simulink library "csbenchlab_est"  (R2024a)
settings: Solver=VariableStepAuto  StartTime=0.0  StopTime=10.0  RelTol=1e-3
undefined symbols (not defined in the file or in its folder): PropagateState_data, PropagateState_DT, PropagateState_params, PropagateState_PT
settings Model: Creator=luka  LastModifiedBy=luka

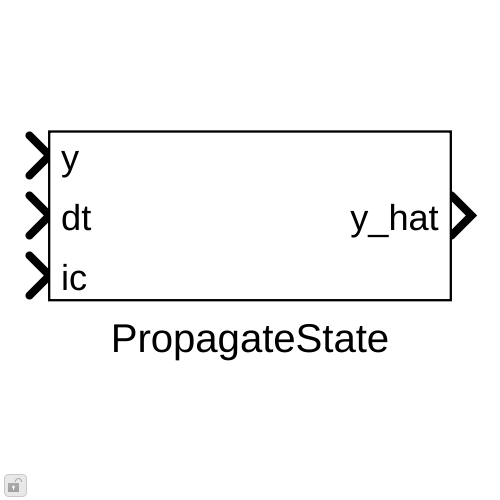
[thumbnail: Simulink's stored preview of the top-level diagram]
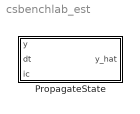
== system csbenchlab_est ==
  PropagateState : Subsystem  Tag=__cs_m_est;  mask{params=PropagateState_params, data=PropagateState_data, ParamsType=PropagateState_PT, DataType=PropagateState_DT}
      mask prompts: params "Parameter struct:"

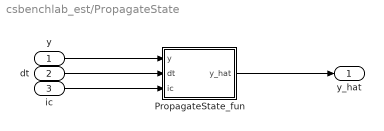
== system csbenchlab_est/PropagateState ==
  y : Inport
  dt : Inport  Port=2
  ic : Inport  Port=3
  PropagateState_fun : MATLAB Function  TreatAsAtomicUnit=on
  y_hat : Outport
  wires:
  y/1 -> PropagateState_fun/1(y)
  dt/1 -> PropagateState_fun/2(dt)
  ic/1 -> PropagateState_fun/3(ic)
  PropagateState_fun/1(y_hat) -> y_hat/1

== matlab function csbenchlab_est/PropagateState/PropagateState_fun ==
  settings: updateMethod=DISCRETE
  data: y input; y_hat output; dt input; ic input; data parameter DataType; params parameter ParamsType
% __classname:=PropagateState;
function y_hat = fcn(y, dt, ic, data, params)
  persistent obj
  if isempty(obj)
    obj = PropagateState(params, 'Data', data);
    obj = obj.configure(ic);
  end
 [obj, y_hat] = obj.step(y, dt);
end
